simulink model "Pi_Pi"  (R2015a)
settings: Solver=ode45  StartTime=0.0  StopTime=10.0  RelTol=1e-3
libraries: simulink x2
settings Model: Creator=vitor  LastModifiedBy=vitor

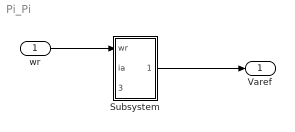
== system Pi_Pi ==
  wr : Inport
  Subsystem : Subsystem
  Varef : Outport
  wires:
  wr/1 -> Subsystem/1(wr)
  Subsystem/1(Varef) -> Varef/1

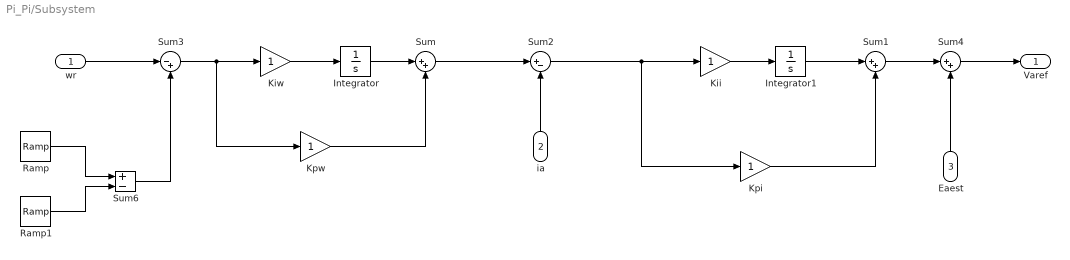
== system Pi_Pi/Subsystem ==
  wr : Inport
  ia : Inport  Port=2
  Eaest : Inport  Port=3
  Integrator : Integrator
  Integrator1 : Integrator
  Kii : Gain
  Kiw : Gain
  Kpi : Gain
  Kpw : Gain
  Ramp : simulink/Sources/Ramp  slope=125  start=0  X0=0
  Ramp1 : simulink/Sources/Ramp  slope=125  start=1  X0=0
  Sum : Sum  Inputs=|++
  Sum1 : Sum  Inputs=|++
  Sum2 : Sum  Inputs=|+-
  Sum3 : Sum  Inputs=|-+
  Sum4 : Sum  Inputs=|++
  Sum6 : Sum  Inputs=+-
  Varef : Outport
  wires:
  Kpw/1 -> Sum/2
  Kii/1 -> Integrator1/1
  Integrator/1 -> Sum/1
  Sum3/1 -> Kpw/1, Kiw/1
  Kpi/1 -> Sum1/2
  wr/1 -> Sum3/1
  ia/1 -> Sum2/2
  Sum1/1 -> Sum4/1
  Sum2/1 -> Kpi/1, Kii/1
  Sum/1 -> Sum2/1
  Integrator1/1 -> Sum1/1
  Kiw/1 -> Integrator/1
  Ramp/1 -> Sum6/1
  Ramp1/1 -> Sum6/2
  Sum6/1 -> Sum3/2
  Eaest/1 -> Sum4/2
  Sum4/1 -> Varef/1
